simulink model "two_phase_boost_converter2"  (R2021a)
settings: Solver=VariableStepAuto  StartTime=0.0  StopTime=0.02  RelTol=1e-3
InitFcn:
  | L=400e-6;
  | C=1000e-6
  | r=0.4
libraries: spsCurrentMeasurementLib x5, simulink x5, spsParallelRLCBranchLib x4, spsSeriesRLCBranchLib x3, dspsigops x3, spsDiodeLib x2, spsMosfetLib x2, spsVoltageMeasurementLib x2, spspowerguiLib x2, spsDCVoltageSourceLib x1
settings Model: Creator=Dell  LastModifiedBy=Dell

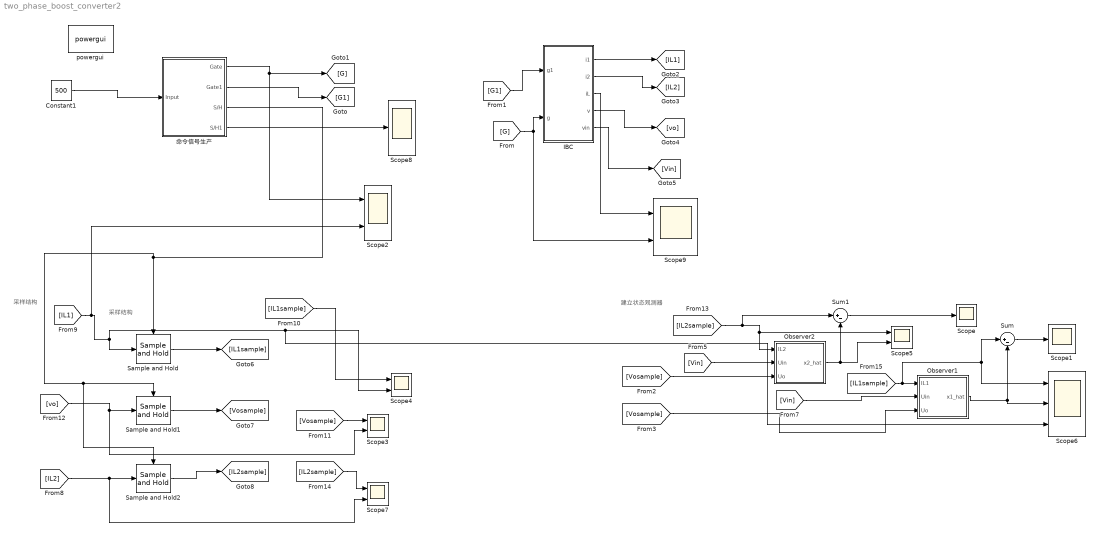
== system two_phase_boost_converter2 ==
  note: 建立状态观测器
  note: 采样结构
  note: 采样结构
  Constant1 : Constant  Value=500
  IBC : Subsystem  mask{Vin=12, C=1000e-6, Load=2, L=400e-6, r=0.4}
  Observer1 : Subsystem
  Observer2 : Subsystem
  Sample and Hold : dspsigops/Sample and Hold  trig=Rising edge  initCond=0  latchinput=off
  Sample and Hold1 : dspsigops/Sample and Hold  trig=Rising edge  initCond=0  latchinput=off
  Sample and Hold2 : dspsigops/Sample and Hold  trig=Rising edge  initCond=0  latchinput=off
  Scope : Scope
  Scope1 : Scope
  Scope{2..5,7,9} (6 alike) : Scope  NumInputPorts=2
  Scope6 : Scope  NumInputPorts=3
  Scope8 : Scope
  Sum : Sum  Inputs=|+-
  Sum1 : Sum  Inputs=|+-
  powergui : spspowerguiLib/powergui  Priority=1  SimulationMode=Discrete  SampleTime=2.5e-6  frequency=60  Iterations=50  frequencyindice=0  Pbase=100e6  ErrMax=1e-4  UnitsV=kV  UnitsW=MW  buscounter=0  FunctionMessages=off  echomessages=off  EnableUseOfTLC=off  CurrentSourceSwitches=on  DisableSnubberDevices=off  DisableRonSwitches=off  DisableVfSwitches=off  DisplayEquations=off  AutomaticDiscreteSolvers=off  SolverType=Tustin  Interpol=off  ExternalGateDelay=off  methode=off  Ts=100  x0status=blocks  SPID=off  SwTol=0  HookPort=off  NonlinearTolerance=1e-4  nMaxIteration=100  ContinueOnMaxIteration=off  RestoreLinks=warning  ResistiveCurrentMeasurement=off  Frange=[0:2:500]  Ylog=off  Xlog=on  ShowGrid=off  save=off  variable=ZData  structure=ScopeData  ZoomFFT=off  StartTime=0.033333  cycles=1  DisplayStyle=1  fundamental=300000  FreqAxis=on  MaxFrequency=300000  frequencyindicesteady=1  RmsSteady=1  display=off
  命令信号生产 : Subsystem  mask{Fs=25e3}
      mask prompts: Fs "swicthing frequency"
  wires:
  IBC/3(iL) -> Scope9/1
  [G] -> IBC/2(g), Scope9/2
  命令信号生产/2(Gate1) -> [G1]
  命令信号生产/1(Gate) -> Scope2/1, [G]
  Constant1/1 -> 命令信号生产/1(Input)
  [G1] -> IBC/1(g1)
  IBC/1(i1) -> [IL1]
  IBC/2(i2) -> [IL2]
  IBC/4(v) -> [vo]
  IBC/5(vin) -> [Vin]
  [IL2sample] -> Sum1/1, Observer2/1(IL2), Scope5/1
  [IL1sample] -> Sum/1, Scope6/1, Observer1/1(IL1)
  [Vin] -> Observer2/2(Uin)
  [Vosample] -> Observer2/3(Uo)
  [Vin] -> Observer1/2(Uin)
  [Vosample] -> Observer1/3(Uo)
  Observer2/1(x2_hat) -> Sum1/2, Scope5/2
  Observer1/1(x1_hat) -> Sum/2, Scope6/2
  Sum/1 -> Scope1/1
  Sample and Hold1/1 -> [Vosample]
  命令信号生产/3(S/H) -> Sample and Hold2/Trigger, Sample and Hold1/Trigger, Sample and Hold/Trigger
  [vo] -> Scope3/2, Sample and Hold1/1
  Sample and Hold/1 -> [IL1sample]
  [Vosample] -> Scope3/1
  [IL1sample] -> Scope4/1
  [IL2sample] -> Scope7/1
  Sample and Hold2/1 -> [IL2sample]
  [IL2] -> Scope7/2, Sample and Hold2/1
  命令信号生产/4(S/H1) -> Scope8/1
  [IL1] -> Scope2/2, Scope6/3, Scope4/2, Sample and Hold/1
  Sum1/1 -> Scope/1

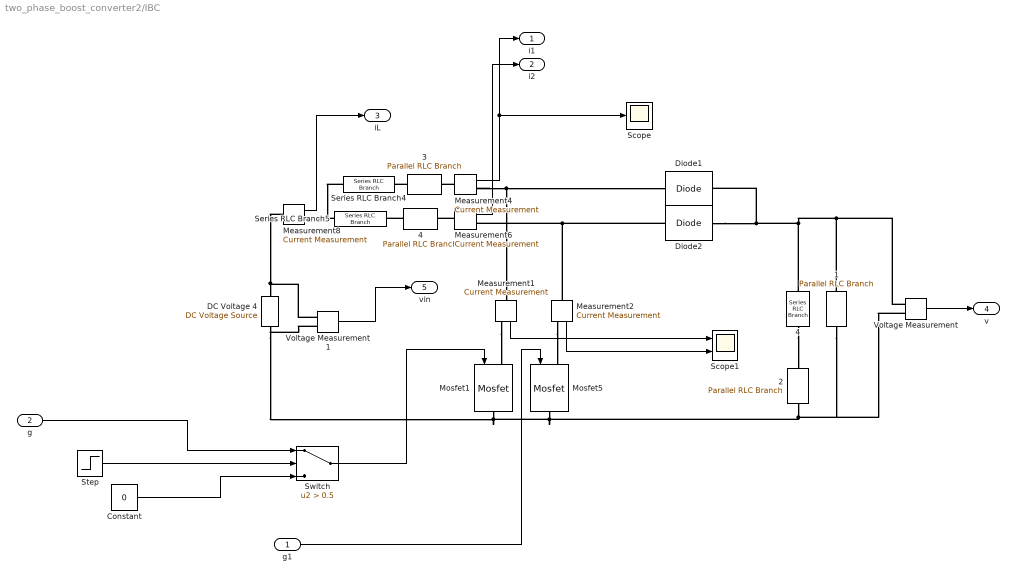
== system two_phase_boost_converter2/IBC ==
  g1 : Inport
  g : Inport  Port=2
  "    4" : spsSeriesRLCBranchLib/Series RLC Branch  LConnTagsString=__new0  RConnTagsString=__new0  BranchType=C  Resistance=0  Inductance=69e-3  SetiL0=off  InitialCurrent=0  Capacitance=C  Setx0=off  InitialVoltage=0  Measurements=None
  "  1" : spsParallelRLCBranchLib/Parallel RLC Branch  LConnTagsString=a  RConnTagsString=__new0  BranchType=R  Resistance=Load  Inductance=1e-3  SetiL0=off  InitialCurrent=0  Capacitance=1e-6  Setx0=off  InitialVoltage=0  Measurements=None
  "  2" : spsParallelRLCBranchLib/Parallel RLC Branch  LConnTagsString=a  RConnTagsString=__new0  BranchType=R  Resistance=0.04  Inductance=1e-3  SetiL0=off  InitialCurrent=0  Capacitance=1e-6  Setx0=off  InitialVoltage=0  Measurements=None
  "  3" : spsParallelRLCBranchLib/Parallel RLC Branch  LConnTagsString=a  RConnTagsString=__new0  BranchType=R  Resistance=r  Inductance=1e-3  SetiL0=off  InitialCurrent=0  Capacitance=1e-6  Setx0=off  InitialVoltage=0  Measurements=None
  "  4" : spsParallelRLCBranchLib/Parallel RLC Branch  LConnTagsString=a  RConnTagsString=__new0  BranchType=R  Resistance=r  Inductance=1e-3  SetiL0=off  InitialCurrent=0  Capacitance=1e-6  Setx0=off  InitialVoltage=0  Measurements=None
   Measurement{1..2,4,6,8} (5 alike) : spsCurrentMeasurementLib/Current Measurement  PhasorSimulation=off  OutputType=Complex  PSBequivalent=0
  Constant : Constant  Value=0
  DC Voltage 4 : spsDCVoltageSourceLib/DC Voltage Source  Amplitude=Vin  Measurements=Voltage
  Diode1 : spsDiodeLib/Diode  Ron=0.001  Lon=0  Vf=0.8  IC=0  UseSnubber=off  Rs=inf  Cs=250e-9  Measurements=off
  Diode2 : spsDiodeLib/Diode  Ron=0.001  Lon=0  Vf=0.8  IC=0  UseSnubber=off  Rs=inf  Cs=250e-9  Measurements=off
  Mosfet1 : spsMosfetLib/Mosfet  Ron=0.1  Lon=0  Rd=0.01  Vfd=0  IC=0  Rs=1e5  Cs=inf  Measurements=off
  Mosfet5 : spsMosfetLib/Mosfet  Ron=0.1  Lon=0  Rd=0.01  Vfd=0  IC=0  Rs=1e5  Cs=inf  Measurements=off
  Scope : Scope
  Scope1 : Scope  NumInputPorts=2
  Series RLC Branch4 : spsSeriesRLCBranchLib/Series RLC Branch  LConnTagsString=__new0  RConnTagsString=__new0  BranchType=L  Resistance=0  Inductance=L  SetiL0=off  InitialCurrent=0  Capacitance=1e-6  Setx0=off  InitialVoltage=0  Measurements=None
  Series RLC Branch5 : spsSeriesRLCBranchLib/Series RLC Branch  LConnTagsString=__new0  RConnTagsString=__new0  BranchType=L  Resistance=0  Inductance=L  SetiL0=off  InitialCurrent=0  Capacitance=1e-6  Setx0=off  InitialVoltage=0  Measurements=None
  Step : Step  Time=0.01  Before=1  After=0  SampleTime=0
  Switch : Switch  Criteria=u2 > Threshold  Threshold=0.5
  Voltage Measurement : spsVoltageMeasurementLib/Voltage Measurement  PhasorSimulation=off  OutputType=Complex  PSBequivalent=0
  Voltage Measurement1 : spsVoltageMeasurementLib/Voltage Measurement  PhasorSimulation=off  OutputType=Complex  PSBequivalent=0
  i1 : Outport
  i2 : Outport  Port=2
  iL : Outport  Port=3
  v : Outport  Port=4
  vin : Outport  Port=5
  wires:
  " Measurement4"/1 -> Scope/1, i1/1
  " Measurement8"/1 -> iL/1
  " Measurement6"/1 -> i2/1
  Voltage Measurement/1 -> v/1
  Step/1 -> Switch/2
  " Measurement1"/1 -> Scope1/1
  " Measurement2"/1 -> Scope1/2
  g/1 -> Switch/1
  Constant/1 -> Switch/3
  g1/1 -> Mosfet5/1
  Switch/1 -> Mosfet1/1
  Voltage Measurement1/1 -> vin/1
  connections:
  Diode2/LConn1 -- " Measurement2"/LConn1 -- " Measurement6"/RConn1
  " Measurement8"/LConn1 -- Voltage Measurement1/LConn1 -- DC Voltage 4/RConn1
  "  2"/RConn1 -- Voltage Measurement/LConn2 -- "  1"/RConn1 -- Mosfet5/RConn1 -- Voltage Measurement1/LConn2 -- DC Voltage 4/LConn1 -- Mosfet1/RConn1
  Series RLC Branch4/LConn1 -- Series RLC Branch5/LConn1 -- " Measurement8"/RConn1
  " Measurement4"/LConn1 -- "  3"/LConn1
  " Measurement6"/LConn1 -- "  4"/LConn1
  Voltage Measurement/LConn1 -- "    4"/LConn1 -- Diode2/RConn1 -- Diode1/RConn1 -- "  1"/LConn1
  " Measurement4"/RConn1 -- " Measurement1"/LConn1 -- Diode1/LConn1
  " Measurement1"/RConn1 -- Mosfet1/LConn1
  " Measurement2"/RConn1 -- Mosfet5/LConn1
  "    4"/RConn1 -- "  2"/LConn1
  "  3"/RConn1 -- Series RLC Branch4/RConn1
  "  4"/RConn1 -- Series RLC Branch5/RConn1

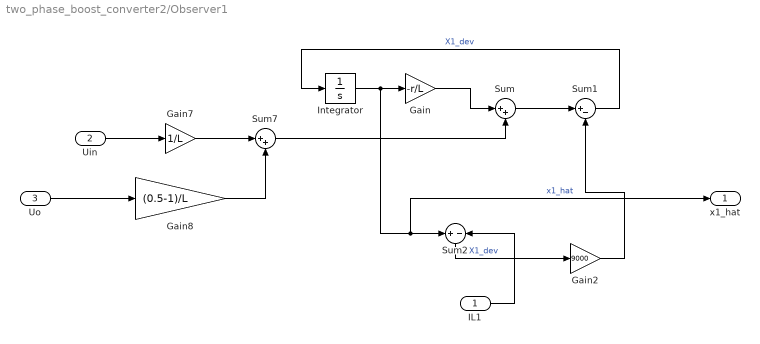
== system two_phase_boost_converter2/Observer1 ==
  IL1 : Inport
  Uin : Inport  Port=2
  Uo : Inport  Port=3
  Gain : Gain  Gain=-r/L
  Gain2 : Gain  Gain=9000
  Gain7 : Gain  Gain=1/L
  Gain8 : Gain  Gain=(0.5-1)/L
  Integrator : Integrator
  Sum : Sum  Inputs=|++
  Sum1 : Sum  Inputs=|+-
  Sum2 : Sum  Inputs=+-
  Sum7 : Sum  Inputs=|++
  x1_hat : Outport
  wires:
  Gain/1 -> Sum/1
  Gain2/1 -> Sum1/2
  Sum7/1 -> Sum/2
  Integrator/1 -> Gain/1, x1_hat/1, Sum2/1  "x1_hat"
  Gain7/1 -> Sum7/1
  Sum1/1 -> Integrator/1  "X1_dev"
  Sum2/1 -> Gain2/1  "X1_dev"
  Gain8/1 -> Sum7/2
  Sum/1 -> Sum1/1
  Uin/1 -> Gain7/1
  Uo/1 -> Gain8/1
  IL1/1 -> Sum2/2

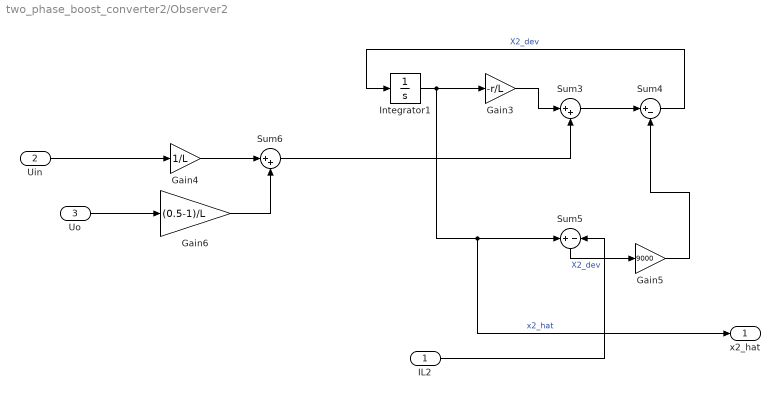
== system two_phase_boost_converter2/Observer2 ==
  IL2 : Inport
  Uin : Inport  Port=2
  Uo : Inport  Port=3
  Gain3 : Gain  Gain=-r/L
  Gain4 : Gain  Gain=1/L
  Gain5 : Gain  Gain=9000
  Gain6 : Gain  Gain=(0.5-1)/L
  Integrator1 : Integrator
  Sum3 : Sum  Inputs=|++
  Sum4 : Sum  Inputs=|+-
  Sum5 : Sum  Inputs=+-
  Sum6 : Sum  Inputs=|++
  x2_hat : Outport
  wires:
  Gain6/1 -> Sum6/2
  Sum4/1 -> Integrator1/1  "X2_dev"
  Sum3/1 -> Sum4/1
  Sum6/1 -> Sum3/2
  Integrator1/1 -> x2_hat/1, Sum5/1, Gain3/1  "x2_hat"
  Gain4/1 -> Sum6/1
  Sum5/1 -> Gain5/1  "X2_dev"
  Gain3/1 -> Sum3/1
  Uo/1 -> Gain6/1
  Gain5/1 -> Sum4/2
  Uin/1 -> Gain4/1
  IL2/1 -> Sum5/2

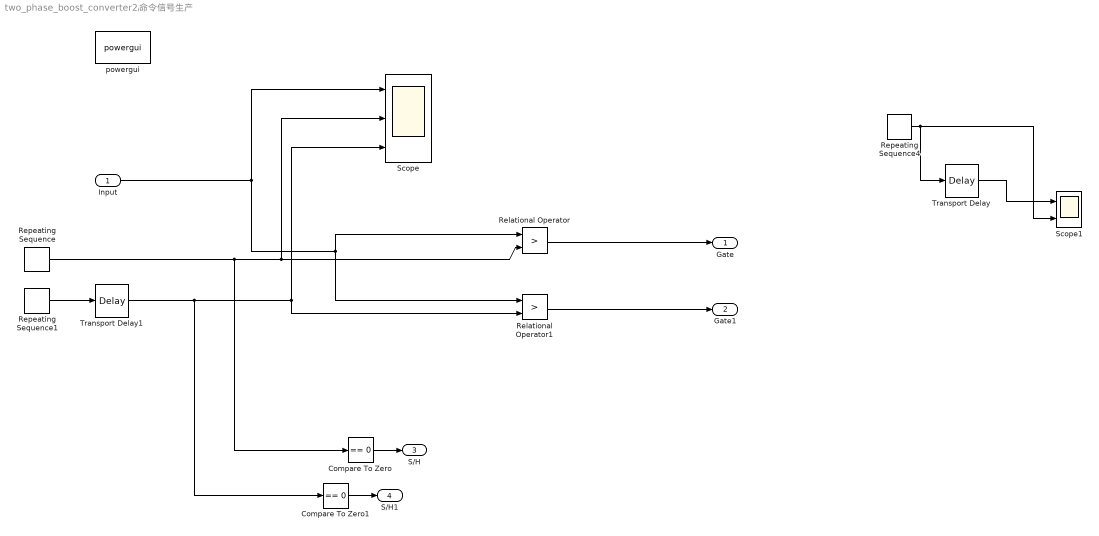
== system two_phase_boost_converter2/命令信号生产 ==
  Input : Inport
  Compare To Zero : simulink/Logic and Bit Operations/Compare To Zero  relop===  OutDataTypeStr=boolean
  Compare To Zero1 : simulink/Logic and Bit Operations/Compare To Zero  relop===  OutDataTypeStr=boolean
  Relational Operator : RelationalOperator  Operator=>  OutDataTypeStr=boolean  RndMeth=Simplest
  Relational Operator1 : RelationalOperator  Operator=>  OutDataTypeStr=boolean  RndMeth=Simplest
  Repeating Sequence : simulink/Sources/Repeating Sequence  rep_seq_t=[0 1./Fs./2 1./Fs]  rep_seq_y=[0 1000 0]
  Repeating Sequence1 : simulink/Sources/Repeating Sequence  rep_seq_t=[0 1./Fs./2 1./Fs]  rep_seq_y=[0 1000 0]
  Repeating Sequence4 : simulink/Sources/Repeating Sequence  rep_seq_t=[0 1./100e3./2 1./100e3]  rep_seq_y=[0 1000 0]
  Scope : Scope  NumInputPorts=3
  Scope1 : Scope  NumInputPorts=2
  Transport Delay : TransportDelay  DelayTime=1./100e3./3
  Transport Delay1 : TransportDelay  DelayTime=1./Fs./2
  powergui : spspowerguiLib/powergui  Priority=1  SimulationMode=Discrete  SampleTime=2.5e-8  frequency=60  Iterations=50  frequencyindice=0  Pbase=100e6  ErrMax=1e-4  UnitsV=kV  UnitsW=MW  buscounter=0  FunctionMessages=off  echomessages=off  EnableUseOfTLC=off  CurrentSourceSwitches=on  DisableSnubberDevices=off  DisableRonSwitches=off  DisableVfSwitches=off  DisplayEquations=off  AutomaticDiscreteSolvers=off  SolverType=Tustin  Interpol=off  ExternalGateDelay=off  methode=off  Ts=100  x0status=blocks  SPID=off  SwTol=0  HookPort=off  NonlinearTolerance=1e-4  nMaxIteration=100  ContinueOnMaxIteration=off  RestoreLinks=warning  ResistiveCurrentMeasurement=off  Frange=[0:2:500]  Ylog=off  Xlog=on  ShowGrid=off  save=off  variable=ZData  structure=ScopeData  ZoomFFT=off  StartTime=0.033333  cycles=1  DisplayStyle=1  fundamental=300000  FreqAxis=on  MaxFrequency=300000  frequencyindicesteady=1  RmsSteady=1  display=off
  Gate : Outport
  Gate1 : Outport  Port=2
  S/H : Outport  Port=3
  S/H1 : Outport  Port=4
  wires:
  Input/1 -> Relational Operator1/1, Relational Operator/1, Scope/1
  Relational Operator/1 -> Gate/1
  Repeating Sequence1/1 -> Transport Delay1/1
  Relational Operator1/1 -> Gate1/1
  Repeating Sequence4/1 -> Transport Delay/1, Scope1/2
  Transport Delay/1 -> Scope1/1
  Repeating Sequence/1 -> Compare To Zero/1, Scope/2, Relational Operator/2
  Compare To Zero/1 -> S/H/1
  Compare To Zero1/1 -> S/H1/1
  Transport Delay1/1 -> Compare To Zero1/1, Relational Operator1/2, Scope/3
